simulink model "untitled"  (Simulink 7.3)
settings: Solver=ode45  StartTime=0.0  StopTime=10.0  RelTol=1e-3
settings Model: Creator=SAINQUAKE  LastModifiedBy=SAINQUAKE
settings DebuggingCC: AlgebraicLoopMsg=none  SolverPrmCheckMsg=none  UnconnectedInputMsg=none  UnconnectedOutputMsg=none  UnconnectedLineMsg=none

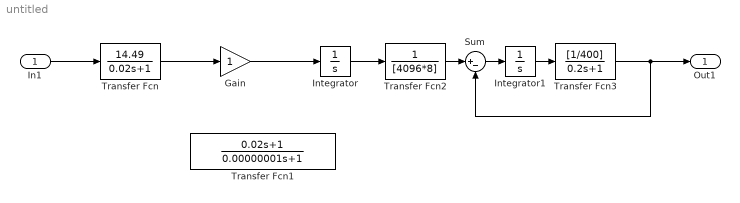
== system untitled ==
  In1 : Inport  OutDataType=fixdt(1, 16)  OutScaling=2^0
  Gain : Gain  ParameterDataType=fixdt(1, 16)  ParameterScaling=2^0  OutDataType=fixdt(1, 16)  OutScaling=2^0
  Integrator : Integrator
  Integrator1 : Integrator
  Sum : Sum  Inputs=|+-  OutDataType=fixdt(1, 16)  OutScaling=2^0
  Transfer Fcn : TransferFcn  Numerator=[14.49]  Denominator=[0.02 1]
  Transfer Fcn1 : TransferFcn  Numerator=[0.02 1]  Denominator=[0.00000001 1]
  Transfer Fcn2 : TransferFcn  Denominator=[4096*8]
  Transfer Fcn3 : TransferFcn  Numerator=[1/400]  Denominator=[0.2 1]
  Out1 : Outport  OutDataType=fixdt(1, 16)  OutScaling=2^0
  wires:
  In1/1 -> Transfer Fcn/1
  Transfer Fcn/1 -> Gain/1
  Integrator/1 -> Transfer Fcn2/1
  Transfer Fcn2/1 -> Sum/1
  Transfer Fcn3/1 -> Out1/1, Sum/2
  Integrator1/1 -> Transfer Fcn3/1
  Sum/1 -> Integrator1/1
  Gain/1 -> Integrator/1
